simulink model "sedemo_outputswitch"  (Simulink 7.5)
settings: Solver=VariableStepDiscrete  StartTime=0.0  StopTime=10.0  RelTol=1e-3
libraries: simeventssink1 x4, simeventsserver1 x1, simeventsrouting1 x1, simeventsattributes2 x1, simeventsgenerators1 x1
settings Model: Creator=The MathWorks Inc.  ExtModeAutoUpdateStatusClock=off
settings DataIOCC: SaveOutput=off  SaveTime=off
settings OptimizationCC: InitFltsAndDblsToZero=on
settings DebuggingCC: SaveWithParameterizedLinksMsg=none  SignalResolutionControl=TryResolveAllWithWarning  SolverPrmCheckMsg=none  MultiTaskDSMMsg=warning  MultiTaskCondExecSysMsg=none  SigSpecEnsureSampleTimeMsg=none  StrictBusMsg=None
settings RTWCC: IncludeERTFirstTime=on
settings GRTTargetCC: TargetFcnLib=ansi_tfl_tmw.mat
settings SimEventsCC: propIdentEventSeed=12345678  propDiagAttribOutput=1  propDiagFcnCallOutput=1  propDiagStatOutput=0

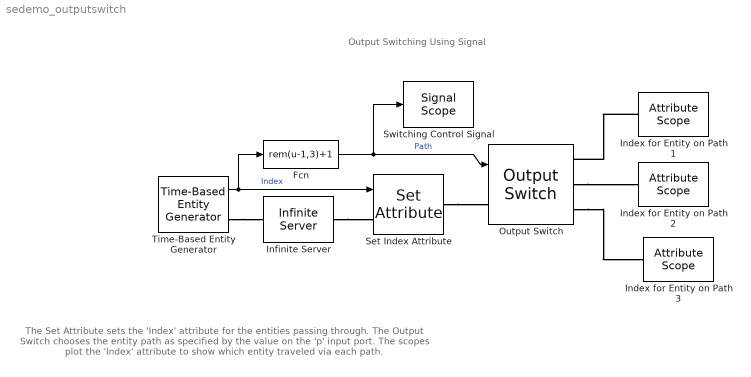
== system sedemo_outputswitch ==
  note: Output Switching Using Signal
  note: The Set Attribute sets the 'Index' attribute for the entities passing through.
      | The Output Switch chooses the entity path as specified by the value on the
      |  'p' input port.  The scopes plot the 'Index' attribute to show which entity
      | traveled via each path.
  Fcn : Fcn  Expr=rem(u-1,3)+1
  Index for Entity on Path 1 : simeventssink1/Attribute Scope  Priority=1  SystemSampleTime=-1  PlotType=Stair  InputType=Attribute  NumInputs=1  AttributeNameY=Index  XInputOptionSignal=Event time  XInputOptionEntity=Event time  AttributeNameX=Count  EnableEntityOutport=off  XMin=0  XMax=10  XLimitExceededOption=Stretch axis limits  YLimitExceededOption=Stretch axis limits  AxisGrid=on  AxisLegend=off  LineDisables=""  LineColors=b  LineStyles=-  LineMarkers=o  OpenScopeAtSimStart=on  Title='Index' for Entity on Path 1  YLabel=Index  XLabel=Time  FigurePosition=[627 540 320 157]  AxisZoom=off  DataStoreOption=Limited  DataPointsLimit=10000  StatNumberArrived=Off  ShowCountPlotted=off  ShowToolbar=on
      settings: YMin=0  YMax=10
  Index for Entity on Path 2 : simeventssink1/Attribute Scope  Priority=1  SystemSampleTime=-1  PlotType=Stair  InputType=Attribute  NumInputs=1  AttributeNameY=Index  XInputOptionSignal=Event time  XInputOptionEntity=Event time  AttributeNameX=Count  EnableEntityOutport=off  XMin=0  XMax=10  XLimitExceededOption=Stretch axis limits  YLimitExceededOption=Stretch axis limits  AxisGrid=on  AxisLegend=off  LineDisables=""  LineColors=b  LineStyles=-  LineMarkers=o  OpenScopeAtSimStart=on  Title='Index' for Entity on Path 2  YLabel=Index  XLabel=Time  FigurePosition=[627 300 320 165]  AxisZoom=off  DataStoreOption=Limited  DataPointsLimit=10000  StatNumberArrived=Off  ShowCountPlotted=off  ShowToolbar=on
      settings: YMin=0  YMax=10
  Index for Entity on Path 3 : simeventssink1/Attribute Scope  Priority=1  SystemSampleTime=-1  PlotType=Stair  InputType=Attribute  NumInputs=1  AttributeNameY=Index  XInputOptionSignal=Event time  XInputOptionEntity=Event time  AttributeNameX=Count  EnableEntityOutport=off  XMin=0  XMax=10  XLimitExceededOption=Stretch axis limits  YLimitExceededOption=Stretch axis limits  AxisGrid=on  AxisLegend=off  LineDisables=""  LineColors=b  LineStyles=-  LineMarkers=o  OpenScopeAtSimStart=on  Title='Index' for Entity on Path 3  YLabel=Index  XLabel=Time  FigurePosition=[626 62 321 164]  AxisZoom=off  DataStoreOption=Limited  DataPointsLimit=10000  StatNumberArrived=Off  ShowCountPlotted=off  ShowToolbar=on
      settings: YMin=0  YMax=10
  Infinite Server : simeventsserver1/Infinite Server  Priority=1  SystemSampleTime=-1  ServiceTimeFrom=Dialog  ServiceTime=0.5  AttributeName=ServiceTime  PriorityServiceCompletion=300  EnableTOPort=off  StatNumberDeparted=Off  StatNumberInBlock=Off  StatPendingEntity=Off  StatNumberPending=Off  StatAverageWait=Off  StatNumberTimedout=Off
  Output Switch : simeventsrouting1/Output Switch  Priority=1  SystemSampleTime=-1  NumberOutputPorts=3  SwitchingCriterion=From signal port p  InitialSeed=34567  AttributeName=Attribute1  InitialConditionsOpt=off  InitialConditions=1  EntityBufferOpt=off  SpecifyEventPriority=on  PriorityOutputSwitchSelectPort=1  TimeoutPortOpt=off  StatNumberDeparted=Off  StatNumberTimedOut=Off  StatPendingEntity=Off  StatLastDeparturePort=Off  EvaluatedNumPorts=3
  Set Index Attribute : simeventsattributes2/Set Attribute  Priority=1  DialogController=des_ddg_create  DialogControllerArgs=DataTag6  SystemSampleTime=-1  AttributeFrom=Signal port  AttributeName=Index  AttributeTreatAsVector=1  AttributeValue=1  AttributeCreate=on  StatNumberDeparted=Off  EvaluatedAttributeValue={[]}
  Switching Control Signal : simeventssink1/Signal Scope  Priority=1  SystemSampleTime=-1  PlotType=Stair  InputType=Signal  NumInputs=1  AttributeNameY=Count  XInputOptionSignal=Event time  XInputOptionEntity=Event time  AttributeNameX=Count  EnableEntityOutport=on  XMin=0  XMax=10  XLimitExceededOption=Stretch axis limits  YLimitExceededOption=Stretch axis limits  AxisGrid=on  AxisLegend=off  LineDisables=""  LineColors=b  LineStyles=-  LineMarkers=.  OpenScopeAtSimStart=on  Title=Switching Control Signal  YLabel=Path  XLabel=Time  FigurePosition=[240 62 379 164]  AxisZoom=off  DataStoreOption=Limited  DataPointsLimit=10000  StatNumberArrived=Off  ShowCountPlotted=off  ShowToolbar=on
      settings: YMin=0  YMax=4
  Time-Based Entity Generator : simeventsgenerators1/Entity Generators/Time-Based Entity Generator  Priority=1  DialogController=des_ddg_create  DialogControllerArgs=DataTag9  SystemSampleTime=-1  GenerateEntitiesUpon=Intergeneration time from dialog  Distribution=Constant  Minimum=0  Maximum=1  Mean=1  InitialSeed=12345  Period=1  PriorityEntityGeneration=500  GenerateEntityAtSimulationStart=off  ResponseWhenBlocked=Pause generation  ResponseWhenUnblocked=Immediate restart  EntityType=Standard  StatNumberDeparted=On  StatPendingEntity=Off  StatAverageIntergenerationTime=Off
  wires:
  Fcn/1 -> Switching Control Signal/1, Output Switch/1  "Path"
  Time-Based Entity Generator/1 -> Fcn/1, Set Index Attribute/1  "Index"
  connections:
  Index for Entity on Path 1/LConn1 -- Output Switch/RConn1
  Output Switch/RConn2 -- Index for Entity on Path 2/LConn1
  Output Switch/RConn3 -- Index for Entity on Path 3/LConn1
  Set Index Attribute/RConn1 -- Output Switch/LConn1
  Time-Based Entity Generator/RConn1 -- Infinite Server/LConn1
  Infinite Server/RConn1 -- Set Index Attribute/LConn1
